simulink model "analyze"  (R2014a)
settings: Solver=FixedStepDiscrete  StartTime=0.0  StopTime=1  FixedStep=0.02  RelTol=1e-3
InitFcn:
  | Veh_Par_wxt
values from neighbouring files (symbols this model uses):
  ag_thr = 0.4*g    (= 3.924)    [Veh_Par_wxt.m]
  B = 2.25    [Veh_Par_wxt.m]
  bra_pre_em = 12    [Veh_Par_wxt.m]
  bra_pre_gz2 = 12/3    (= 4)    [Veh_Par_wxt.m]
  bra_pre_gz34 = 12/3    (= 4)    [Veh_Par_wxt.m]
  bra_pre_yd = 12/2    (= 6)    [Veh_Par_wxt.m]
  brakepre_dem_data = [0 1 2 3 4 5 6 7 8 9 10 11 12]    [Veh_Par_wxt.m]
  brakeTrq_dem_data = [0 218.198 436.396 654.594 872.792 1090.99 1309.188 1527.386 1745.584 1963.782 2181.98 2400.178 2618.376]    [Veh_Par_wxt.m]
  bratrq_max = 4*2618.376    (= 10473.504)    [Veh_Par_wxt.m]
  eff_tran = 0.75    [Veh_Par_wxt.m]
  G = Mass*g    (= 36297)    [Veh_Par_wxt.m]
  kd1 = 1    [Veh_Par_wxt.m]
  kd2 = 1    [Veh_Par_wxt.m]
  kd3 = 1    [Veh_Par_wxt.m]
  ki1 = 1    [Veh_Par_wxt.m]
  ki2 = 1    [Veh_Par_wxt.m]
  ki3 = 1    [Veh_Par_wxt.m]
  kp1 = 1    [Veh_Par_wxt.m]
  kp2 = 1    [Veh_Par_wxt.m]
  kp3 = 1    [Veh_Par_wxt.m]
  L = 3.12    [Veh_Par_wxt.m]
  premax = 12    [Veh_Par_wxt.m]
  Radius = 0.20    (= 0.2)    [Veh_Par_wxt.m]
  s_opt_yi_add = 0.05    [Veh_Par_wxt.m]
  s_opt_zhuan_add = 0.05    [Veh_Par_wxt.m]
  spd_map_mot = [0 100 200 300 360 400 500 600 700 800 900]*tras_ratio    [Veh_Par_wxt.m]
  spdmax = 900*tras_ratio    (= 5580)    [Veh_Par_wxt.m]
  speed_thr_park = 5/3.6/Radius*30/pi    (= 66.3145596216)    [Veh_Par_wxt.m]
  tras_ratio = 6.2    [Veh_Par_wxt.m]
  trq_map_mot = [1200 1200 1200 1200 1200 1080 864 720 617 540 480]/tras_ratio    [Veh_Par_wxt.m]
  trqmax = 80    [Veh_Par_wxt.m]
  v_thr1_b = 5    [Veh_Par_wxt.m]
  v_thr2_b = 20    [Veh_Par_wxt.m]
  v_thr_park = 5    [Veh_Par_wxt.m]
undefined symbols (not defined in the file or in its folder): DiscIntNeverNeededParam
libraries: simulink x231, ec5744lib x19
(part 16 of 16)

== system analyze/MainControl/mode_control/forward/forward/Drive/驱动防滑控制TCS/转向TCS/左转/无滑转 ==
  trq_dem_lf : Inport
  trq_dem_lr : Inport  Port=2
  trq_dem_rf : Inport  Port=3
  trq_dem_rr : Inport  Port=4
  bra_pre_l : Inport  Port=5
  bra_pre_r : Inport  Port=6
  brake_dem : Inport  Port=7
  Action Port : ActionPort  ActionType=case
  1-D Lookup Table : Lookup_n-D  NumberOfTableDimensions=1  BreakpointsForDimension1=brakeTrq_dem_data  Table=brakepre_dem_data  InternalRulePriority=Speed  RndMeth=Simplest  InputSameDT=on
  1-D Lookup Table2 : Lookup_n-D  NumberOfTableDimensions=1  BreakpointsForDimension1=brakeTrq_dem_data  Table=brakepre_dem_data  InternalRulePriority=Speed  RndMeth=Simplest  InputSameDT=on
  Add : Sum
  Add2 : Sum
  Constant : Constant  Value=bratrq_max
  Gain1 : Gain  Gain=1/2
  Gain2 : Gain  Gain=1/100
  Gain3 : Gain  Gain=1/2
  Gain4 : Gain  Gain=1/2
  HeartBeat : MATLAB Function  TreatAsAtomicUnit=on
  HeartBeat1 : MATLAB Function  TreatAsAtomicUnit=on
  Memory : Memory  InheritSampleTime=on
  Memory1 : Memory  InheritSampleTime=on
  Mux : Mux  Inputs=8
  Mux1 : Mux  Inputs=8
  Mux2 : Mux  Inputs=7
  Mux3 : Mux  Inputs=7
  Product : Product
  Saturation{,1..3} (4 alike) : Saturate  UpperLimit=trqmax  LowerLimit=-trqmax
  Saturation4 : Saturate  UpperLimit=premax  LowerLimit=0
  Saturation5 : Saturate  UpperLimit=premax  LowerLimit=0
  SpdLim_dem{,1..3} (4 alike) : Constant  Value=spdmax
  SpdSet_dem{,1..3} (4 alike) : Constant
  TrqLim_dem{,1..3} (4 alike) : Constant
  mot_drive : Constant
  mot_drive1 : Constant  Value=2
  mot_drive2 : Constant
  mot_drive3 : Constant  Value=2
  mot_enable{,1..3} (4 alike) : Constant  Value=2
  mot_mode{,1..3} (4 alike) : Constant
  mot_lf : Outport
  mot_lr : Outport  Port=2
  mot_rf : Outport  Port=3
  mot_rr : Outport  Port=4
  bra_pre_l1 : Outport  Port=5
  bra_pre_r1 : Outport  Port=6
  wires:
  mot_drive/1 -> Mux/3
  mot_mode/1 -> Mux/2
  trq_dem_lf/1 -> Saturation/1
  mot_enable/1 -> Mux/1
  SpdSet_dem/1 -> Mux/5
  Mux/1 -> mot_lf/1
  TrqLim_dem/1 -> Mux/6
  HeartBeat/1(life) -> Mux/8, Memory/1
  Memory/1 -> HeartBeat/1(life_pre)
  SpdLim_dem/1 -> Mux/7
  mot_drive1/1 -> Mux2/3
  mot_mode2/1 -> Mux2/2
  trq_dem_rf/1 -> Saturation2/1
  mot_enable2/1 -> Mux2/1
  SpdSet_dem1/1 -> Mux2/5
  Mux2/1 -> mot_rf/1
  TrqLim_dem1/1 -> Mux2/6
  SpdLim_dem1/1 -> Mux2/7
  mot_drive2/1 -> Mux1/3
  mot_mode1/1 -> Mux1/2
  trq_dem_lr/1 -> Saturation1/1
  mot_enable1/1 -> Mux1/1
  SpdSet_dem2/1 -> Mux1/5
  Mux1/1 -> mot_lr/1
  TrqLim_dem2/1 -> Mux1/6
  HeartBeat1/1(life) -> Mux1/8, Memory1/1
  Memory1/1 -> HeartBeat1/1(life_pre)
  SpdLim_dem2/1 -> Mux1/7
  mot_drive3/1 -> Mux3/3
  mot_mode3/1 -> Mux3/2
  trq_dem_rr/1 -> Saturation3/1
  mot_enable3/1 -> Mux3/1
  SpdSet_dem3/1 -> Mux3/5
  Mux3/1 -> mot_rr/1
  TrqLim_dem3/1 -> Mux3/6
  SpdLim_dem3/1 -> Mux3/7
  bra_pre_l/1 -> Add/2
  Add/1 -> Saturation4/1
  1-D Lookup Table/1 -> Add/1
  Constant/1 -> Product/1
  Product/1 -> Gain1/1
  Gain1/1 -> Gain4/1, Gain3/1
  Gain2/1 -> Product/2
  Gain3/1 -> 1-D Lookup Table/1
  Gain4/1 -> 1-D Lookup Table2/1
  1-D Lookup Table2/1 -> Add2/1
  bra_pre_r/1 -> Add2/2
  Add2/1 -> Saturation5/1
  brake_dem/1 -> Gain2/1
  Saturation/1 -> Mux/4
  Saturation1/1 -> Mux1/4
  Saturation2/1 -> Mux2/4
  Saturation3/1 -> Mux3/4
  Saturation4/1 -> bra_pre_l1/1
  Saturation5/1 -> bra_pre_r1/1

== matlab function analyze/MainControl/mode_control/Park/park/HeartBeat ==
  data: life_pre input; life output
function life = fcn(life_pre)
%#codegen
life=life_pre+1;
if life>15
    life=0;
end
end

== matlab function analyze/MainControl/mode_switch/mode_switch ==
  data: mode_dem input; mode_dem_out output; brake_emerg input; speed_act_lf input; speed_act_lr input; speed_act_rf input; speed_act_rr input; v_act input; v_thr_park input; speed_thr_park input; mode_dem_out_pre input
function mode_dem_out = fcn(mode_dem,brake_emerg,speed_act_lf,speed_act_lr,speed_act_rf,speed_act_rr,v_act,v_thr_park,speed_thr_park,mode_dem_out_pre)
%#codegen
mode_dem_out=mode_dem_out_pre;

if mode_dem==0 && abs(v_act)<=v_thr_park && speed_act_lf<=speed_thr_park && speed_act_lr<=speed_thr_park && speed_act_rf<=speed_thr_park && speed_act_rr<=speed_thr_park && brake_emerg==0
    mode_dem_out=0;
elseif mode_dem==1 && v_act>=-v_thr_park && speed_act_lf>=0 && speed_act_lr>=0 && speed_act_rf>=0 && speed_act_rr>=0 && brake_emerg==0
    mode_dem_out=1;
elseif mode_dem==2 && brake_emerg==0
    mode_dem_out=2;
elseif mode_dem==3 && v_act<=v_thr_park && speed_act_lf>=0 && speed_act_lr>=0 && speed_act_rf>=0 && speed_act_rr>=0 && brake_emerg==0
    mode_dem_out=3;
elseif mode_dem==4 && v_act<=v_thr_park &&  v_act>=-v_thr_park % && speed_act_lf==0 && speed_act_lr==0 && speed_act_rf==0 && speed_act_rr==0 && brake_emerg==0       
    mode_dem_out=4;
elseif brake_emerg==1
    mode_dem_out=5;
% else
%     mode_dem_out=5;
end
end

== matlab function analyze/MainControl/mode_control/Park/park/HeartBeat1 ==
  data: life_pre input; life output
function life = fcn(life_pre)
%#codegen
life=life_pre+1;
if life>15
    life=0;
end
end

== matlab function analyze/MainControl/mode_control/forward/forward/Drive/目标转向力矩确定模块/MATLAB Function ==
  data: steer_dem input; Rturn_min output; G input; L input; umax input; B input; Tpeak_L input; Tpeak_R input; eff_tran input; Radius input; f input
function Rturn_min = fcn(steer_dem,G,L,umax,B,Tpeak_L,Tpeak_R,eff_tran,Radius,f)
%#codegen
if steer_dem>0
    Rturn_min=(G*L*umax/(4*B*(Tpeak_R*eff_tran/Radius-f*G/2))-0.925)/0.15*B;
else
    Rturn_min=(G*L*umax/(4*B*(Tpeak_L*eff_tran/Radius-f*G/2))-0.925)/0.15*B;
end
end

== matlab function analyze/MainControl/mode_control/forward/forward/Drive/目标转向力矩确定模块/MATLAB Function1 ==
  data: v_act input; Rturn_min_ag output; ag_thr input
function Rturn_min_ag = fcn(v_act,ag_thr)
%#codegen

    Rturn_min_ag=(v_act/3.6)^2/ag_thr;
end

== matlab function analyze/MainControl/mode_control/forward/forward/Drive/目标转向力矩确定模块/MATLAB Function2 ==
  data: umax input; delta_Tsteer_max output; G input; L input; B input; Radius input; Rturn_min_xy input
function delta_Tsteer_max = fcn(umax,G,L,B,Radius,Rturn_min_xy)
%#codegen

    delta_Fsteer_max=umax/(0.925+0.15*(Rturn_min_xy/B))*G*L/(2*B);
    delta_Tsteer_max=delta_Fsteer_max*Radius;
    
end

== matlab function analyze/MainControl/mode_control/forward/forward/Drive/MATLAB Function ==
  data: acc_y input; y output; steer_dem input; ag_thr input
function y = fcn(acc_y,steer_dem,ag_thr)
%#codegen
if abs(acc_y)>=ag_thr
    y=0;
elseif steer_dem~=0
    y=1;
else 
    y=2;
end
end

== matlab function analyze/MainControl/mode_control/forward/forward/Drive/左右侧电机分配及功率限制/MATLAB Function ==
  data: trqlim_l input; trq_dem_l output; trq_dem_r output; trq_dem_l1 input; trqlim_r input; trq_dem_r1 input; delta_T_dem input
function [trq_dem_l,trq_dem_r] = fcn(trqlim_l,trq_dem_l1,trqlim_r,trq_dem_r1,delta_T_dem)
%#codegen
if trq_dem_l1==trqlim_l
    trq_dem_l=trq_dem_l1;
    trq_dem_r=trq_dem_l1+delta_T_dem;%这时候加的是负值
elseif trq_dem_r1==trqlim_r
    trq_dem_l=trq_dem_r1-delta_T_dem;
    trq_dem_r=trq_dem_r1;
    
else
    trq_dem_l=trq_dem_l1;
    trq_dem_r=trq_dem_r1;
end
% trq_dem_l=max(0,trq_dem_l);%限一下最小值，不要小于0
% trq_dem_r=max(0,trq_dem_r);
trq_dem_l=max(-trqlim_l,trq_dem_l);%小转向半径下，内侧履带是可能输出负转矩的，从地面吸收功率，给外侧，所以不能限到0，限到最大电机外特性负值
trq_dem_r=max(-trqlim_r,trq_dem_r);
end

== matlab function analyze/MainControl/mode_control/forward/forward/Drive/容错控制/MATLAB Function ==
  data: trq_dem_l input; trq_dem_lf output; trq_dem_r input; trqlim_lf input; trqlim_lr input; trqlim_rf input; trqlim_rr input; guzhang_lf input; guzhang_lr input; guzhang_rf input; guzhang_rr input; trq_dem_lr output; trq_dem_rf output; trq_dem_rr output; bra_pre_l output; bra_pre_r output; bra_pre_gz2 input; bra_pre_gz34 input; mode output
function [trq_dem_lf,trq_dem_lr,trq_dem_rf,trq_dem_rr,bra_pre_l,bra_pre_r,mode] = fcn(trq_dem_l,trq_dem_r,trqlim_lf,trqlim_lr,trqlim_rf,trqlim_rr,guzhang_lf,guzhang_lr,guzhang_rf,guzhang_rr,bra_pre_gz2,bra_pre_gz34)
%#codegen
if guzhang_lf==0 && guzhang_lr==0 && guzhang_rf==0 && guzhang_rr==0    %0电机故障,平均分配
    trq_dem_lf=trq_dem_l/2;
    trq_dem_lr=trq_dem_l/2;
    trq_dem_rf=trq_dem_r/2;
    trq_dem_rr=trq_dem_r/2;
    bra_pre_l=0;
    bra_pre_r=0;
    mode=1;
elseif  guzhang_lf==1 && guzhang_lr==0 && guzhang_rf==0 && guzhang_rr==0  %1电机故障，同侧电机进行力矩转移，超过限值后，对侧亦降扭。
    trq_dem_lf=0;
    trq_dem_lr=min(trq_dem_l,trqlim_lr);
    trq_dem_rf=(trq_dem_r-(trq_dem_l-trq_dem_lr))/2;
    trq_dem_rr=(trq_dem_r-(trq_dem_l-trq_dem_lr))/2;
    bra_pre_l=0;
    bra_pre_r=0;
    mode=2;
elseif  guzhang_lf==0 && guzhang_lr==1 && guzhang_rf==0 && guzhang_rr==0
    trq_dem_lf=min(trq_dem_l,trqlim_lf);
    trq_dem_lr=0;
    trq_dem_rf=(trq_dem_r-(trq_dem_l-trq_dem_lf))/2;
    trq_dem_rr=(trq_dem_r-(trq_dem_l-trq_dem_lf))/2;
    bra_pre_l=0;
    bra_pre_r=0;
    mode=3;
elseif  guzhang_lf==0 && guzhang_lr==0 && guzhang_rf==1 && guzhang_rr==0
    trq_dem_rf=0;
    trq_dem_rr=min(trq_dem_r,trqlim_rr);
    trq_dem_lf=(trq_dem_l-(trq_dem_r-trq_dem_rr))/2;
    trq_dem_lr=(trq_dem_l-(trq_dem_r-trq_dem_rr))/2;
    bra_pre_l=0;
    bra_pre_r=0;
    mode=4;
elseif  guzhang_lf==0 && guzhang_lr==0 && guzhang_rf==0 && guzhang_rr==1
    trq_dem_rf=min(trq_dem_r,trqlim_rf);
    trq_dem_rr=0;
    trq_dem_lf=(trq_dem_l-(trq_dem_r-trq_dem_rf))/2;
    trq_dem_lr=(trq_dem_l-(trq_dem_r-trq_dem_rf))/2;
    bra_pre_l=0;
    bra_pre_r=0;
    mode=5;
elseif  (guzhang_lf==1 && guzhang_lr==1 && guzhang_rf==0 && guzhang_rr==0) || (guzhang_lf==0 && guzhang_lr==0 && guzhang_rf==1 && guzhang_rr==1) %2电机故障，同侧电机故障,电机目标力矩全部置0，并施加制动直至停车
    trq_dem_rf=0;
    trq_dem_rr=0;
    trq_dem_lf=0;
    trq_dem_lr=0;
    bra_pre_l=bra_pre_gz2;
    bra_pre_r=bra_pre_gz2;
    mode=6;
elseif  guzhang_lf==1 && guzhang_lr==0 && guzhang_rf==1 && guzhang_rr==0 %2电机故障，对侧双电机故障,有4种情况,前两电机故障
    trq_dem_lf=0;
    trq_dem_rf=0;
    if trq_dem_l>=trq_dem_r
        trq_dem_lr=min(trq_dem_l,trqlim_lr);
        trq_dem_rr=min(min(trq_dem_r,trqlim_rr),(trq_dem_r-(trq_dem_l-trq_dem_lr)));
    else
        trq_dem_rr=min(trq_dem_r,trqlim_rr);
        trq_dem_lr=min(min(trq_dem_l,trqlim_lr),(trq_dem_l-(trq_dem_r-trq_dem_rr)));
    end
    bra_pre_l=0;
    bra_pre_r=0;
    mode=8;
elseif  guzhang_lf==0 && guzhang_lr==1 && guzhang_rf==0 && guzhang_rr==1 %后两电机故障
    trq_dem_lr=0;
    trq_dem_rr=0;
    if trq_dem_l>=trq_dem_r
        trq_dem_lf=min(trq_dem_l,trqlim_lf);
        trq_dem_rf=min(min(trq_dem_r,trqlim_rf),(trq_dem_r-(trq_dem_l-trq_dem_lf)));
    else
        trq_dem_rf=min(trq_dem_r,trqlim_rf);
        trq_dem_lf=min(min(trq_dem_l,trqlim_lf),(trq_dem_l-(trq_dem_r-trq_dem_rf)));
    end
    bra_pre_l=0;
    bra_pre_r=0;
    mode=9;
elseif  guzhang_lf==1 && guzhang_lr==0 && guzhang_rf==0 && guzhang_rr==1 %左前电机和右后电机故障
    trq_dem_lf=0;
    trq_dem_rr=0;
    if trq_dem_l>=trq_dem_r
        trq_dem_lr=min(trq_dem_l,trqlim_lr);
        trq_dem_rf=min(min(trq_dem_r,trqlim_rf),(trq_dem_r-(trq_dem_l-trq_dem_lr)));
    else
        trq_dem_rf=min(trq_dem_r,trqlim_rf);
        trq_dem_lr=min(min(trq_dem_l,trqlim_lr),(trq_dem_l-(trq_dem_r-trq_dem_rf)));
    end
    bra_pre_l=0;
    bra_pre_r=0;
    mode=10;
elseif  guzhang_lf==0 && guzhang_lr==1 && guzhang_rf==1 && guzhang_rr==0 %左后电机和右前电机故障
    trq_dem_lr=0;
    trq_dem_rf=0;
    if trq_dem_l>=trq_dem_r
        trq_dem_lf=min(trq_dem_l,trqlim_lf);
        trq_dem_rr=min(min(trq_dem_r,trqlim_rr),(trq_dem_r-(trq_dem_l-trq_dem_lf)));
    else
        trq_dem_rr=min(trq_dem_r,trqlim_rr);
        trq_dem_lf=min(min(trq_dem_l,trqlim_lf),(trq_dem_l-(trq_dem_r-trq_dem_rr)));
    end
    bra_pre_l=0;
    bra_pre_r=0;
    mode=11;
else
    %     (guzhang_lf==1 && guzhang_lr==1 && guzhang_rf==1 && guzhang_rr==0) || (guzhang_lf==1 && guzhang_lr==1 && guzhang_rf==0 && guzhang_rr==1) || (guzhang_lf==1 && guzhang_lr==0 && guzhang_rf==1 && guzhang_rr==1) || (guzhang_lf==0 && guzhang_lr==1 && guzhang_rf==1 && guzhang_rr==1) || (guzhang_lf==1 && guzhang_lr==1 && guzhang_rf==1 && guzhang_rr==1)
    % 三电机或者四电机故障
    trq_dem_rf=0;
    trq_dem_rr=0;
    trq_dem_lf=0;
    trq_dem_lr=0;
    bra_pre_l=bra_pre_gz34;
    bra_pre_r=bra_pre_gz34;
    mode=12;
end
% trq_dem_lf=max(0,trq_dem_lf);%电机转矩不小于0，就是不能出现负值
% trq_dem_lr=max(0,trq_dem_lr);
% trq_dem_rf=max(0,trq_dem_rf);
% trq_dem_rr=max(0,trq_dem_rr);
trq_dem_lf=max(-trqlim_lf,trq_dem_lf);%电机转矩可以出现负值，不超过负的外特性
trq_dem_lr=max(-trqlim_lr,trq_dem_lr);
trq_dem_rf=max(-trqlim_rf,trq_dem_rf);
trq_dem_rr=max(-trqlim_rr,trq_dem_rr);
bra_pre_l=bra_pre_l;
bra_pre_r=bra_pre_r;
end

== matlab function analyze/MainControl/mode_control/forward/forward/Drive/驱动防滑控制TCS/MATLAB Function ==
  data: steer_dem input; y output
function y = fcn(steer_dem)
%#codegen 如果有转向，y=0,无转向，y=1
if steer_dem~=0
y = 0;
else y=1;
end
end

== matlab function analyze/MainControl/mode_control/forward/forward/Drive/驱动防滑控制TCS/转向TCS/MATLAB Function ==
  data: steer_dem input; y output
function y = fcn(steer_dem)
%#codegen左转为0，右转为1
if steer_dem>0
    y=0;
else
    y = 1;
end
end

== matlab function analyze/MainControl/mode_control/forward/forward/Drive/驱动防滑控制TCS/转向TCS/左转/MATLAB Function ==
  data: s_act_lf input; flag_lf output; s_opt_zhuan input; s_opt_zhuan_add input; flag_lf_pre input
function flag_lf = fcn(s_act_lf,s_opt_zhuan,s_opt_zhuan_add,flag_lf_pre)
%#codegen
if s_act_lf>s_opt_zhuan+s_opt_zhuan_add
    flag_lf=1;
elseif s_act_lf<s_opt_zhuan
    flag_lf = 0;
else
    flag_lf=flag_lf_pre;
end
end

== matlab function analyze/MainControl/mode_control/forward/forward/Drive/驱动防滑控制TCS/转向TCS/左转/MATLAB Function1 ==
  data: s_act_lr input; flag_lr output; s_opt_zhuan input; s_opt_zhuan_add input; flag_lr_pre input
function flag_lr = fcn(s_act_lr,s_opt_zhuan,s_opt_zhuan_add,flag_lr_pre)
%#codegen
if s_act_lr>s_opt_zhuan+s_opt_zhuan_add
    flag_lr=1;
elseif s_act_lr<s_opt_zhuan
    flag_lr = 0;
else
    flag_lr=flag_lr_pre;
end
end

== matlab function analyze/MainControl/mode_control/forward/forward/Drive/驱动防滑控制TCS/转向TCS/左转/MATLAB Function2 ==
  data: s_act_rf input; flag_rf output; s_opt_zhuan input; s_opt_zhuan_add input; flag_rf_pre input
function flag_rf = fcn(s_act_rf,s_opt_zhuan,s_opt_zhuan_add,flag_rf_pre)
%#codegen
if s_act_rf>s_opt_zhuan+s_opt_zhuan_add
    flag_rf=1;
elseif s_act_rf<s_opt_zhuan
    flag_rf = 0;
else
    flag_rf=flag_rf_pre;
end
end

== matlab function analyze/MainControl/mode_control/forward/forward/Drive/驱动防滑控制TCS/转向TCS/左转/MATLAB Function3 ==
  data: s_act_rr input; flag_rr output; s_opt_zhuan input; s_opt_zhuan_add input; flag_rr_pre input
function flag_rr = fcn(s_act_rr,s_opt_zhuan,s_opt_zhuan_add,flag_rr_pre)
%#codegen
if s_act_rr>s_opt_zhuan+s_opt_zhuan_add
    flag_rr=1;
elseif s_act_rr<s_opt_zhuan
    flag_rr = 0;
else
    flag_rr=flag_rr_pre;
end
end

== matlab function analyze/MainControl/mode_control/forward/forward/Drive/驱动防滑控制TCS/转向TCS/左转/MATLAB Function4 ==
  data: y output; flag_rf input; flag_rr input
function y = fcn(flag_rf,flag_rr)
%#codegen只判断外侧车轮滑转状况，不能满足要求再进一步修改。
if flag_rf==0 && flag_rr==0
    y=0;
elseif flag_rf==1 && flag_rr==0
    y=1;
elseif flag_rf==0 && flag_rr==1
    y=2;
else
    %     flag_rf==1 && flag_rr==1
    y=3;
end
end

== matlab function analyze/MainControl/mode_control/forward/forward/Drive/驱动防滑控制TCS/转向TCS/左转/无滑转/HeartBeat ==
  data: life_pre input; life output
function life = fcn(life_pre)
%#codegen
life=life_pre+1;
if life>15
    life=0;
end
end

== matlab function analyze/MainControl/mode_control/forward/forward/Drive/驱动防滑控制TCS/转向TCS/左转/无滑转/HeartBeat1 ==
  data: life_pre input; life output
function life = fcn(life_pre)
%#codegen
life=life_pre+1;
if life>15
    life=0;
end
end

== matlab function analyze/MainControl/mode_control/forward/forward/Drive/驱动防滑控制TCS/转向TCS/左转/前轮滑转/HeartBeat ==
  data: life_pre input; life output
function life = fcn(life_pre)
%#codegen
life=life_pre+1;
if life>15
    life=0;
end
end

== matlab function analyze/MainControl/mode_control/forward/forward/Drive/驱动防滑控制TCS/转向TCS/左转/前轮滑转/HeartBeat1 ==
  data: life_pre input; life output
function life = fcn(life_pre)
%#codegen
life=life_pre+1;
if life>15
    life=0;
end
end

== matlab function analyze/MainControl/mode_control/forward/forward/Drive/驱动防滑控制TCS/转向TCS/左转/后轮滑转/HeartBeat ==
  data: life_pre input; life output
function life = fcn(life_pre)
%#codegen
life=life_pre+1;
if life>15
    life=0;
end
end

== matlab function analyze/MainControl/mode_control/forward/forward/Drive/驱动防滑控制TCS/转向TCS/左转/后轮滑转/HeartBeat1 ==
  data: life_pre input; life output
function life = fcn(life_pre)
%#codegen
life=life_pre+1;
if life>15
    life=0;
end
end

== matlab function analyze/MainControl/mode_control/forward/forward/Drive/驱动防滑控制TCS/转向TCS/左转/前后轮均滑转/HeartBeat ==
  data: life_pre input; life output
function life = fcn(life_pre)
%#codegen
life=life_pre+1;
if life>15
    life=0;
end
end

== matlab function analyze/MainControl/mode_control/forward/forward/Drive/驱动防滑控制TCS/转向TCS/左转/前后轮均滑转/HeartBeat1 ==
  data: life_pre input; life output
function life = fcn(life_pre)
%#codegen
life=life_pre+1;
if life>15
    life=0;
end
end

== matlab function analyze/MainControl/mode_control/forward/forward/Drive/驱动防滑控制TCS/转向TCS/右转/MATLAB Function ==
  data: s_act_lf input; flag_lf output; s_opt_zhuan input; s_opt_zhuan_add input; flag_lf_pre input
function flag_lf = fcn(s_act_lf,s_opt_zhuan,s_opt_zhuan_add,flag_lf_pre)
%#codegen
if s_act_lf>s_opt_zhuan+s_opt_zhuan_add
    flag_lf=1;
elseif s_act_lf<s_opt_zhuan
    flag_lf = 0;
else
    flag_lf=flag_lf_pre;
end
end

== matlab function analyze/MainControl/mode_control/forward/forward/Drive/驱动防滑控制TCS/转向TCS/右转/MATLAB Function1 ==
  data: s_act_lr input; flag_lr output; s_opt_zhuan input; s_opt_zhuan_add input; flag_lr_pre input
function flag_lr = fcn(s_act_lr,s_opt_zhuan,s_opt_zhuan_add,flag_lr_pre)
%#codegen
if s_act_lr>s_opt_zhuan+s_opt_zhuan_add
    flag_lr=1;
elseif s_act_lr<s_opt_zhuan
    flag_lr = 0;
else
    flag_lr=flag_lr_pre;
end
end

== matlab function analyze/MainControl/mode_control/forward/forward/Drive/驱动防滑控制TCS/转向TCS/右转/MATLAB Function2 ==
  data: s_act_rf input; flag_rf output; s_opt_zhuan input; s_opt_zhuan_add input; flag_rf_pre input
function flag_rf = fcn(s_act_rf,s_opt_zhuan,s_opt_zhuan_add,flag_rf_pre)
%#codegen
if s_act_rf>s_opt_zhuan+s_opt_zhuan_add
    flag_rf=1;
elseif s_act_rf<s_opt_zhuan
    flag_rf = 0;
else
    flag_rf=flag_rf_pre;
end
end

== matlab function analyze/MainControl/mode_control/forward/forward/Drive/驱动防滑控制TCS/转向TCS/右转/MATLAB Function3 ==
  data: s_act_rr input; flag_rr output; s_opt_zhuan input; s_opt_zhuan_add input; flag_rr_pre input
function flag_rr = fcn(s_act_rr,s_opt_zhuan,s_opt_zhuan_add,flag_rr_pre)
%#codegen
if s_act_rr>s_opt_zhuan+s_opt_zhuan_add
    flag_rr=1;
elseif s_act_rr<s_opt_zhuan
    flag_rr = 0;
else
    flag_rr=flag_rr_pre;
end
end

== matlab function analyze/MainControl/mode_control/forward/forward/Drive/驱动防滑控制TCS/转向TCS/右转/MATLAB Function4 ==
  data: y output; flag_lf input; flag_lr input
function y = fcn(flag_lf,flag_lr)
%#codegen只判断外侧车轮滑转状况，不能满足要求再进一步修改。
if flag_lf==0 && flag_lr==0
    y=0;
elseif flag_lf==1 && flag_lr==0
    y=1;
elseif flag_lf==0 && flag_lr==1
    y=2;
else
    %     flag_lf==1 && flag_lr==1
    y=3;
end
end

== matlab function analyze/MainControl/mode_control/forward/forward/Drive/驱动防滑控制TCS/转向TCS/右转/前轮滑转/HeartBeat ==
  data: life_pre input; life output
function life = fcn(life_pre)
%#codegen
life=life_pre+1;
if life>15
    life=0;
end
end

== matlab function analyze/MainControl/mode_control/forward/forward/Drive/驱动防滑控制TCS/转向TCS/右转/前轮滑转/HeartBeat1 ==
  data: life_pre input; life output
function life = fcn(life_pre)
%#codegen
life=life_pre+1;
if life>15
    life=0;
end
end

== matlab function analyze/MainControl/mode_control/forward/forward/Drive/驱动防滑控制TCS/转向TCS/右转/后轮滑转/HeartBeat ==
  data: life_pre input; life output
function life = fcn(life_pre)
%#codegen
life=life_pre+1;
if life>15
    life=0;
end
end

== matlab function analyze/MainControl/mode_control/forward/forward/Drive/驱动防滑控制TCS/转向TCS/右转/后轮滑转/HeartBeat1 ==
  data: life_pre input; life output
function life = fcn(life_pre)
%#codegen
life=life_pre+1;
if life>15
    life=0;
end
end

== matlab function analyze/MainControl/mode_control/forward/forward/Drive/驱动防滑控制TCS/转向TCS/右转/前后轮均滑转/HeartBeat ==
  data: life_pre input; life output
function life = fcn(life_pre)
%#codegen
life=life_pre+1;
if life>15
    life=0;
end
end

== matlab function analyze/MainControl/mode_control/forward/forward/Drive/驱动防滑控制TCS/转向TCS/右转/无滑转/HeartBeat ==
  data: life_pre input; life output
function life = fcn(life_pre)
%#codegen
life=life_pre+1;
if life>15
    life=0;
end
end

== matlab function analyze/MainControl/mode_control/forward/forward/MATLAB Function ==
  data: acc_dem input; y output; brake_dem input; HAC input
function y = fcn(acc_dem,brake_dem,HAC)
%#codegen
if HAC==1
    if acc_dem>0
        y=0;
    else
        y=1;
    end
else
    if brake_dem==0
        y=0;
    else
        y=1;
    end
end
end

== matlab function analyze/MainControl/mode_control/neutral/neutral/HeartBeat ==
  data: life_pre input; life output
function life = fcn(life_pre)
%#codegen
life=life_pre+1;
if life>15
    life=0;
end
end

== matlab function analyze/MainControl/mode_control/forward/forward/Brake/MATLAB Function2 ==
  data: syi_act_lr input; flagyi_lr output; s_opt_yi input; s_opt_yi_add input; flagyi_lr_pre input
function flagyi_lr = fcn(syi_act_lr,s_opt_yi,s_opt_yi_add,flagyi_lr_pre)
%#codegen
if syi_act_lr>s_opt_yi+s_opt_yi_add
    flagyi_lr=1;
elseif syi_act_lr<s_opt_yi
    flagyi_lr = 0;
else
    flagyi_lr=flagyi_lr_pre;
end
end

== matlab function analyze/MainControl/mode_control/forward/forward/Brake/MATLAB Function4 ==
  data: syi_act_rr input; flagyi_rr output; s_opt_yi input; s_opt_yi_add input; flagyi_rr_pre input
function flagyi_rr = fcn(syi_act_rr,s_opt_yi,s_opt_yi_add,flagyi_rr_pre)
%#codegen
if syi_act_rr>s_opt_yi+s_opt_yi_add
    flagyi_rr=1;
elseif syi_act_rr<s_opt_yi
    flagyi_rr = 0;
else
    flagyi_rr=flagyi_rr_pre;
end
end

== matlab function analyze/MainControl/mode_control/forward/forward/Brake/HeartBeat1 ==
  data: life_pre input; life output
function life = fcn(life_pre)
%#codegen
life=life_pre+1;
if life>15
    life=0;
end
end

== matlab function analyze/MainControl/mode_control/center_steer/center_steer/容错控制/MATLAB Function ==
  data: trq_dem_l input; trq_dem_lf output; trq_dem_r input; trqlim_lf input; trqlim_lr input; trqlim_rf input; trqlim_rr input; guzhang_lf input; guzhang_lr input; guzhang_rf input; guzhang_rr input; trq_dem_lr output; trq_dem_rf output; trq_dem_rr output; bra_pre_l output; bra_pre_r output; bra_pre_yd input; mode output
function [trq_dem_lf,trq_dem_lr,trq_dem_rf,trq_dem_rr,bra_pre_l,bra_pre_r,mode] = fcn(trq_dem_l,trq_dem_r,trqlim_lf,trqlim_lr,trqlim_rf,trqlim_rr,guzhang_lf,guzhang_lr,guzhang_rf,guzhang_rr,bra_pre_yd)
%#codegen
if guzhang_lf==0 && guzhang_lr==0 && guzhang_rf==0 && guzhang_rr==0    %0电机故障,平均分配
    trq_dem_lf=trq_dem_l/2;
    trq_dem_lr=trq_dem_l/2;
    trq_dem_rf=trq_dem_r/2;
    trq_dem_rr=trq_dem_r/2;
    bra_pre_l=0;
    bra_pre_r=0;
    mode=1;
elseif  guzhang_lf==1 && guzhang_lr==0 && guzhang_rf==0 && guzhang_rr==0  %1电机故障，同侧电机进行力矩转移,跟行车不同，对侧不降扭。
    trq_dem_lf=0;
    trq_dem_lr=min(trq_dem_l,trqlim_lr);
    trq_dem_rf=trq_dem_r/2;
    trq_dem_rr=trq_dem_r/2;
    bra_pre_l=0;
    bra_pre_r=0;
    mode=2;
elseif  guzhang_lf==0 && guzhang_lr==1 && guzhang_rf==0 && guzhang_rr==0
    trq_dem_lf=min(trq_dem_l,trqlim_lf);
    trq_dem_lr=0;
    trq_dem_rf=trq_dem_r/2;
    trq_dem_rr=trq_dem_r/2;
    bra_pre_l=0;
    bra_pre_r=0;
    mode=3;
elseif  guzhang_lf==0 && guzhang_lr==0 && guzhang_rf==1 && guzhang_rr==0
    trq_dem_rf=0;
    trq_dem_rr=min(trq_dem_r,trqlim_rr);
    trq_dem_lf=trq_dem_l/2;
    trq_dem_lr=trq_dem_l/2;
    bra_pre_l=0;
    bra_pre_r=0;
    mode=4;
elseif  guzhang_lf==0 && guzhang_lr==0 && guzhang_rf==0 && guzhang_rr==1
    trq_dem_rf=min(trq_dem_r,trqlim_rf);
    trq_dem_rr=0;
    trq_dem_lf=trq_dem_l/2;
    trq_dem_lr=trq_dem_l/2;
    bra_pre_l=0;
    bra_pre_r=0;
    mode=5;
elseif  guzhang_lf==1 && guzhang_lr==1 && guzhang_rf==0 && guzhang_rr==0  %2电机故障，左侧双电机故障，左侧履带施加制动，改为原地转向
    trq_dem_lf=0;
    trq_dem_lr=0;
    trq_dem_rf=trq_dem_r/2;
    trq_dem_rr=trq_dem_r/2;
    bra_pre_l=bra_pre_yd;
    bra_pre_r=0;
    mode=6;
elseif  guzhang_lf==0 && guzhang_lr==0 && guzhang_rf==1 && guzhang_rr==1  %右侧双电机故障
    trq_dem_lf=trq_dem_l/2;
    trq_dem_lr=trq_dem_l/2;
    trq_dem_rf=0;
    trq_dem_rr=0;
    bra_pre_l=0;
    bra_pre_r=bra_pre_yd;
    mode=7;
elseif  guzhang_lf==1 && guzhang_lr==0 && guzhang_rf==1 && guzhang_rr==0 %2电机故障，对侧双电机故障,有4种情况,前两电机故障
    trq_dem_lf=0;
    trq_dem_rf=0;
    trq_dem_lr=min(trq_dem_l,trqlim_lr);
    trq_dem_rr=min(trq_dem_r,trqlim_rr);
    bra_pre_l=0;
    bra_pre_r=0;
    mode=8;
elseif  guzhang_lf==0 && guzhang_lr==1 && guzhang_rf==0 && guzhang_rr==1 %后两电机故障
    trq_dem_lr=0;
    trq_dem_rr=0;
    trq_dem_lf=min(trq_dem_l,trqlim_lf);
    trq_dem_rf=min(trq_dem_r,trqlim_rf);
    bra_pre_l=0;
    bra_pre_r=0;
    mode=9;
elseif  guzhang_lf==1 && guzhang_lr==0 && guzhang_rf==0 && guzhang_rr==1 %左前电机和右后电机故障
    trq_dem_lf=0;
    trq_dem_rr=0;
    trq_dem_lr=min(trq_dem_l,trqlim_lr);
    trq_dem_rf=min(trq_dem_r,trqlim_rf);
    bra_pre_l=0;
    bra_pre_r=0;
    mode=10;
elseif  guzhang_lf==0 && guzhang_lr==1 && guzhang_rf==1 && guzhang_rr==0 %左后电机和右前电机故障
    trq_dem_lr=0;
    trq_dem_rf=0;
    trq_dem_lf=min(trq_dem_l,trqlim_lf);
    trq_dem_rr=min(trq_dem_r,trqlim_rr);
    bra_pre_l=0;
    bra_pre_r=0;
    mode=11;
elseif guzhang_lf==1 && guzhang_lr==1 && guzhang_rf==1 && guzhang_rr==0   % 三电机故障
    trq_dem_lf=0;
    trq_dem_lr=0;
    trq_dem_rf=0;
    trq_dem_rr=min(trq_dem_r,trqlim_rr);
    bra_pre_l=bra_pre_yd;
    bra_pre_r=0;
    mode=12;
elseif guzhang_lf==1 && guzhang_lr==1 && guzhang_rf==0 && guzhang_rr==1
    trq_dem_lf=0;
    trq_dem_lr=0;
    trq_dem_rf=min(trq_dem_r,trqlim_rf);
    trq_dem_rr=0;
    bra_pre_l=bra_pre_yd;
    bra_pre_r=0;
    mode=13;
elseif guzhang_lf==1 && guzhang_lr==0 && guzhang_rf==1 && guzhang_rr==1
    trq_dem_lf=0;
    trq_dem_lr=min(trq_dem_l,trqlim_lr);
    trq_dem_rf=0;
    trq_dem_rr=0;
    bra_pre_l=0;
    bra_pre_r=bra_pre_yd;
    mode=14;
elseif guzhang_lf==0 && guzhang_lr==1 && guzhang_rf==1 && guzhang_rr==1
    trq_dem_lf=min(trq_dem_l,trqlim_lf);
    trq_dem_lr=0;
    trq_dem_rf=0;
    trq_dem_rr=0;
    bra_pre_l=0;
    bra_pre_r=bra_pre_yd;
    mode=15;
else
    %     guzhang_lf==1 && guzhang_lr==1 && guzhang_rf==1 && guzhang_rr==1 %四电机故障
    trq_dem_lf=0;
    trq_dem_lr=0;
    trq_dem_rf=0;
    trq_dem_rr=0;
    bra_pre_l=0;
    bra_pre_r=0;
    mode=16;
end
trq_dem_lf=min(trqlim_lf,trq_dem_lf);trq_dem_lf=max(0,trq_dem_lf);
trq_dem_lr=min(trqlim_lr,trq_dem_lr);trq_dem_lr=max(0,trq_dem_lr);
trq_dem_rf=min(trqlim_rf,trq_dem_rf);trq_dem_rf=max(0,trq_dem_rf);
trq_dem_rr=min(trqlim_rr,trq_dem_rr);trq_dem_rr=max(0,trq_dem_rr);
bra_pre_l=bra_pre_l;
bra_pre_r=bra_pre_r;
end
